simulink model "trans"  (R2013a)
settings: Solver=ode45  StartTime=0.0  StopTime=100.0  RelTol=1e-3  AbsTol=1e-6
values from neighbouring files (symbols this model uses):
  A = [-a1/A1 0; a1/A2 -a2/A2]    [transmitacje.m]
  B = [1/A1 0; 0 1/A2]    [transmitacje.m]
  C = eye(2)    [transmitacje.m]
  D = zeros(2)    [transmitacje.m]
  dfwew1 = 0.1*fwew1max    [Kaskady.m]    (also in Kaskady2.m = 0; transmitacje.m)
  dfwew2 = 0.1*fwew2max    [Kaskady.m]    (also in Kaskady2.m; transmitacje.m)
  fwew1 = k(i)*fwew1max    [Kaskady.m]    (also in Kaskady2.m = 0.1; transmitacje.m = 0)
  fwew2 = 0.1    [Kaskady.m]    (also in Kaskady2.m = k(i)*fwew2max; transmitacje.m = 0)
  h = [h10 h20]    [transmitacje.m]
  t0 = 1    [Kaskady.m]    (also in Kaskady2.m; Skoki.m = 0; symulek1.m; transmitacje.m)
settings Model: Creator=LAB320-1552  LastModifiedBy=LAB320-1552
settings DebuggingCC: SolverPrmCheckMsg=none

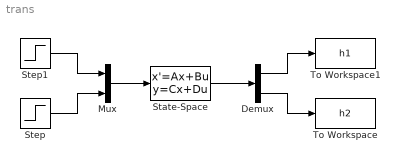
== system trans ==
  Demux : Demux  Outputs=2
  Mux : Mux  Inputs=2
  State-Space : StateSpace  A=A  B=B  C=C  D=D  X0=h
  Step : Step  Time=t0  Before=fwew2  After=fwew2+dfwew2  SampleTime=0
  Step1 : Step  Time=t0  Before=fwew1  After=fwew1+dfwew1  SampleTime=0
  To Workspace : ToWorkspace  VariableName=h2  SampleTime=-1
  To Workspace1 : ToWorkspace  VariableName=h1  SampleTime=-1
  wires:
  Demux/1 -> To Workspace1/1
  Demux/2 -> To Workspace/1
  State-Space/1 -> Demux/1
  Mux/1 -> State-Space/1
  Step1/1 -> Mux/1
  Step/1 -> Mux/2
